simulink model "LADRC_ct"  (R2024b)
settings: Solver=VariableStepAuto  StartTime=0.0  StopTime=10.0  RelTol=1e-3
values from neighbouring files (symbols this model uses):
  A = [zeros(N, 1)  eye(N, N) ... (first row only)    [LADRC_ct_vars.m]
  b = 0.2    [ADRC_playground_vars.m]    (also in LADRC_ct_vars.m = [zeros(N-1, 1))
  b0 = 0.4    [ADRC_playground_vars.m]    (also in LADRC_ct_vars.m = 0.75)
  c_t = [1, zeros(1, N)]    [LADRC_ct_vars.m]
  k = ones(N,1)    [LADRC_ct_vars.m]
  l = ones(N+1, 1)    [LADRC_ct_vars.m]
  N = order(plant)    [LADRC_ct_vars.m]
libraries: simulink x2
settings Model: Creator=Henrik  LastModifiedBy=Henrik

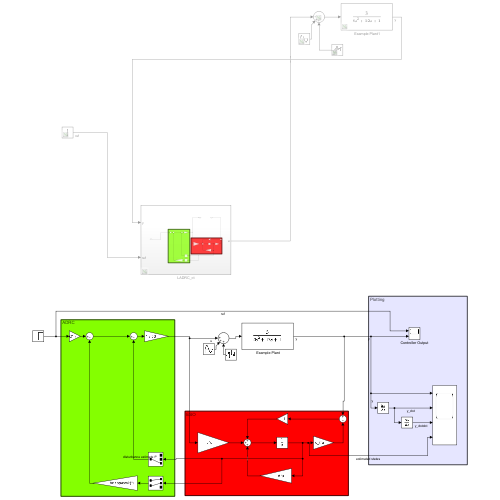
[thumbnail: Simulink's stored preview of the top-level diagram]
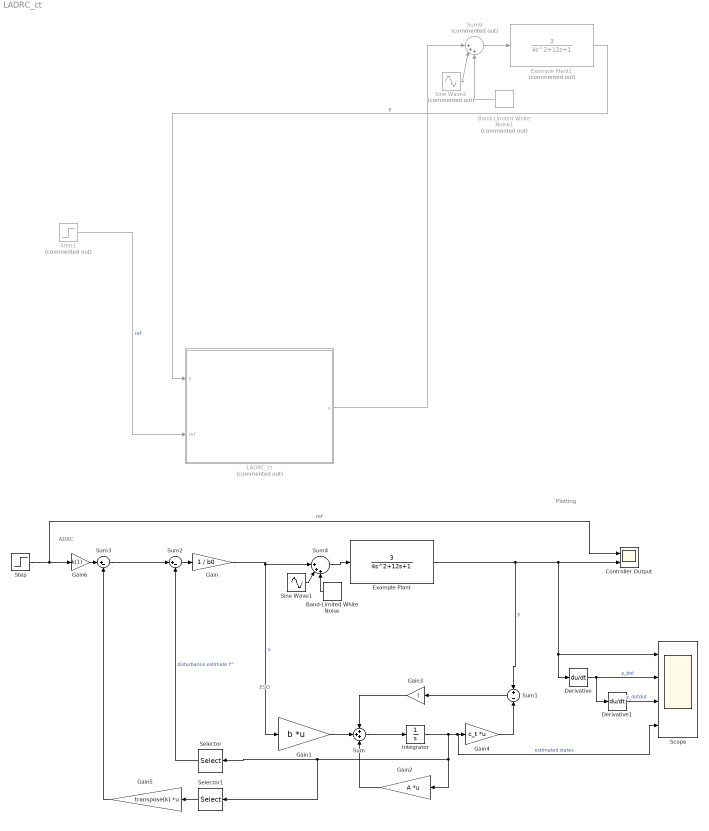
== system LADRC_ct ==
  note: ADRC
  note: ESO
  note: Plotting
  " Example Plant" : TransferFcn  Numerator=[3]  Denominator=[4 12 1]
  " Example Plant1" : TransferFcn  Commented=on  Numerator=[3]  Denominator=[4 12 1]
  Band-Limited White Noise : simulink/Sources/Band-Limited White Noise  Cov=[0]  Ts=0.01  seed=[23341]
  Band-Limited White Noise1 : simulink/Sources/Band-Limited White Noise  Commented=on  Cov=[1]  Ts=0.01  seed=[23341]
  Controller Output : Scope  NumInputPorts=2
  Derivative : Derivative
  Derivative1 : Derivative
  Gain : Gain  Gain=1 / b0
  Gain1 : Gain  Gain=b  Multiplication=Matrix(K*u)
  Gain2 : Gain  Gain=A  Multiplication=Matrix(K*u)
  Gain3 : Gain  Gain=l
  Gain4 : Gain  Gain=c_t  Multiplication=Matrix(K*u)
  Gain5 : Gain  Gain=transpose(k)  Multiplication=Matrix(K*u)
  Gain6 : Gain  Gain=k(1)
  Integrator : Integrator
  LADRC_ct : Subsystem  Commented=on
  Scope : Scope  NumInputPorts=4
  Selector : Selector  InputPortWidth=N+1  IndexOptions=Index vector (dialog)  Indices=[N+1]  OutputSizes=1
  Selector1 : Selector  InputPortWidth=N+1  IndexOptions=Index vector (dialog)  Indices=[1:N]  OutputSizes=1
  Sine Wave1 : Sin  Amplitude=0  Frequency=60  SampleTime=0
  Sine Wave2 : Sin  Commented=on  Amplitude=2  Frequency=60  SampleTime=0
  Step : Step  SampleTime=0
  Step1 : Step  Commented=on  SampleTime=0
  Sum : Sum  Inputs=+++
  Sum1 : Sum  Inputs=+|-
  Sum2 : Sum  Inputs=|+-
  Sum3 : Sum  Inputs=|+-
  Sum4 : Sum  Inputs=||+++
  Sum9 : Sum  Commented=on  Inputs=||+++
  wires:
  Gain/1 -> Sum4/1, Gain1/1  "u"
  Gain1/1 -> Sum/2
  Sum/1 -> Integrator/1
  Gain2/1 -> Sum/3
  Sum1/1 -> Gain3/1
  Gain3/1 -> Sum/1
  Gain4/1 -> Sum1/2
  Integrator/1 -> Scope/4, Gain4/1, Gain2/1, Selector1/1, Selector/1  "estimated states"
  Sum2/1 -> Gain/1
  Selector/1 -> Sum2/2  "disturbance estimate f^"
  Selector1/1 -> Gain5/1
  Gain5/1 -> Sum3/2
  Step/1 -> Controller Output/1, Gain6/1  "ref"
  Gain6/1 -> Sum3/1
  Sum3/1 -> Sum2/1
  Derivative/1 -> Derivative1/1, Scope/2  "y_dot"
  Derivative1/1 -> Scope/3  "y_dotdot"
  Sum4/1 -> " Example Plant"/1
  Sine Wave1/1 -> Sum4/2
  Band-Limited White Noise/1 -> Sum4/3
  Band-Limited White Noise1/1 -> Sum9/3
  Sine Wave2/1 -> Sum9/2
  Sum9/1 -> " Example Plant1"/1
  " Example Plant1"/1 -> LADRC_ct/1(y)  "y"
  Step1/1 -> LADRC_ct/2(ref)  "ref"
  LADRC_ct/1(u) -> Sum9/1
  " Example Plant"/1 -> Sum1/1, Derivative/1, Scope/1, Controller Output/2  "y"

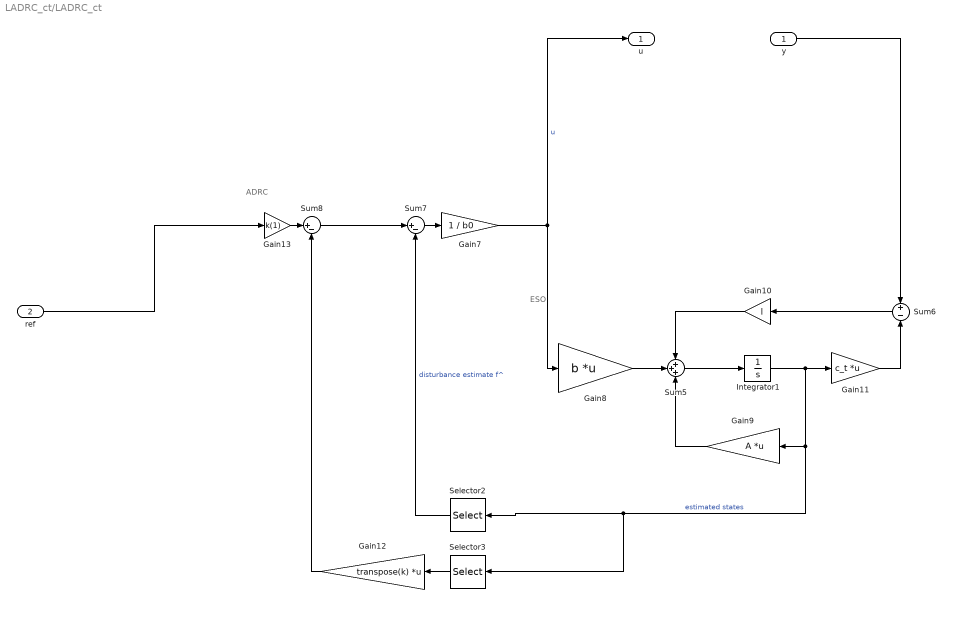
== system LADRC_ct/LADRC_ct ==
  note: ESO
  note: ADRC
  y : Inport
  ref : Inport  Port=2
  Gain10 : Gain  Gain=l
  Gain11 : Gain  Gain=c_t  Multiplication=Matrix(K*u)
  Gain12 : Gain  Gain=transpose(k)  Multiplication=Matrix(K*u)
  Gain13 : Gain  Gain=k(1)
  Gain7 : Gain  Gain=1 / b0
  Gain8 : Gain  Gain=b  Multiplication=Matrix(K*u)
  Gain9 : Gain  Gain=A  Multiplication=Matrix(K*u)
  Integrator1 : Integrator
  Selector2 : Selector  InputPortWidth=N+1  IndexOptions=Index vector (dialog)  Indices=[N+1]  OutputSizes=1
  Selector3 : Selector  InputPortWidth=N+1  IndexOptions=Index vector (dialog)  Indices=[1:N]  OutputSizes=1
  Sum5 : Sum  Inputs=+++
  Sum6 : Sum  Inputs=+|-
  Sum7 : Sum  Inputs=|+-
  Sum8 : Sum  Inputs=|+-
  u : Outport
  wires:
  Gain8/1 -> Sum5/2
  Gain7/1 -> u/1, Gain8/1  "u"
  Integrator1/1 -> Gain11/1, Selector3/1, Selector2/1, Gain9/1  "estimated states"
  Gain11/1 -> Sum6/2
  Sum6/1 -> Gain10/1
  Selector2/1 -> Sum7/2  "disturbance estimate f^"
  Sum7/1 -> Gain7/1
  Gain12/1 -> Sum8/2
  Gain10/1 -> Sum5/1
  Gain9/1 -> Sum5/3
  Gain13/1 -> Sum8/1
  Sum5/1 -> Integrator1/1
  Selector3/1 -> Gain12/1
  Sum8/1 -> Sum7/1
  ref/1 -> Gain13/1
  y/1 -> Sum6/1
